simulink model "simple_control"  (R2018a)
settings: Solver=VariableStepAuto  StartTime=0.0  StopTime=10.0  RelTol=1e-3
settings Model: Creator=Kim  LastModifiedBy=Kim

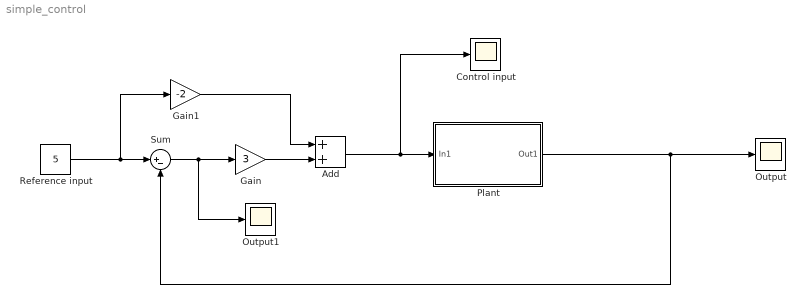
== system simple_control ==
  Add : Sum
  Control input : Scope
  Gain : Gain  Gain=3
  Gain1 : Gain  Gain=-2
  Output : Scope
  Output1 : Scope
  Plant : Subsystem
  Reference input : Constant  Value=5
  Sum : Sum  Inputs=|+-
  wires:
  Plant/1(Out1) -> Output/1, Sum/2
  Reference input/1 -> Sum/1, Gain1/1
  Sum/1 -> Output1/1, Gain/1
  Gain/1 -> Add/2
  Gain1/1 -> Add/1
  Add/1 -> Control input/1, Plant/1(In1)

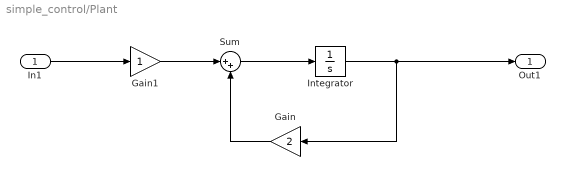
== system simple_control/Plant ==
  In1 : Inport
  Gain : Gain  Gain=2
  Gain1 : Gain
  Integrator : Integrator
  Sum : Sum  Inputs=|++
  Out1 : Outport
  wires:
  Sum/1 -> Integrator/1
  Integrator/1 -> Out1/1, Gain/1
  In1/1 -> Gain1/1
  Gain/1 -> Sum/2
  Gain1/1 -> Sum/1
